simulink model "mbed_disco_F407_usbSerial"  (R2015a)
settings: Solver=FixedStepDiscrete  SolverMode=SingleTasking  StartTime=0.0  StopTime=10.0  FixedStep=1  RelTol=1e-3
libraries: mbed_lib x3, mbed_targets_stm_disco_f429 x1
settings Model: Creator=Stuv  LastModifiedBy=Stuv
settings OptimizationCC: OptimizeModelRefInitCode=on  LifeSpan=1
settings HardwareCC: ProdLargestAtomicInteger=Long  ProdLargestAtomicFloat=Double  ProdEndianess=LittleEndian  ProdHWDeviceType=ARM Compatible->ARM Cortex
settings RTWCC: SystemTargetFile=mbed.tlc  TemplateMakefile=mbed.tmf  Description=Mbed Target (Embedded Target)  TargetLang=C++
settings CodeAppCC: IgnoreCustomStorageClasses=off
settings STFCustomTargetCC: CombineOutputUpdateFcns=on  SupportContinuousTime=off  SupportVariableSizeSignals=off  SystemTargetFile=mbed.tlc
settings ERTTargetCC: SupportContinuousTime=off  SupportVariableSizeSignals=off  ERTCustomFileTemplate=mbed_file_process.tlc

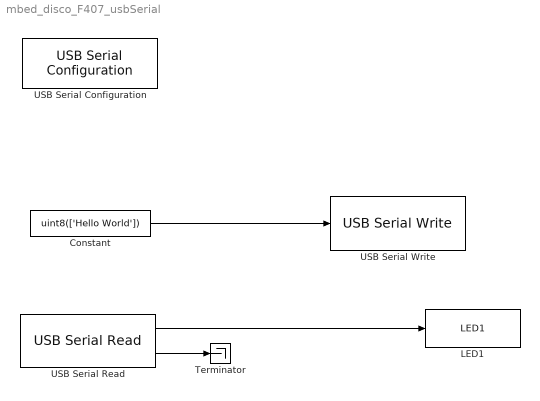
== system mbed_disco_F407_usbSerial ==
  Constant : Constant  Value=uint8(['Hello World'])
  LED1 : mbed_targets_stm_disco_f429/LED1  Parameter1=0
  Terminator : Terminator
  USB Serial Configuration : mbed_lib/Serial/USB Serial Configuration
  USB Serial Read : mbed_lib/Serial/USB Serial Read  PortWidth=1  SampleTime=-1
  USB Serial Write : mbed_lib/Serial/USB Serial Write  numData=off  SampleTime=-1
  wires:
  Constant/1 -> USB Serial Write/1
  USB Serial Read/2 -> Terminator/1
  USB Serial Read/1 -> LED1/1
